simulink model "sm_tractor_row_crop"  (R2024b)
settings: Solver=ode23t  StartTime=0.0  StopTime=20  FixedStep=1/1000  MaxStep=0.2  RelTol=1e-3  AbsTol=1e-3  EnableMultiTasking=on
PostLoadFcn:
  | sm_tractor_row_crop_config_maneuver(bdroot,VehicleData,'stepsteer');
StartFcn:
  | tic
StopFcn:
  | Elapsed_Sim_Time = toc;
undefined symbols (not defined in the file): FL, FR, HMPST, InitVehicle, Maneuver, RL, RR, SceneData, targetSpeed, VehicleData, X, Y, Z
libraries: sm_lib x84, sm_vehicle_utilities_lib x40, fl_lib x15, nesl_utility x14, simulink x4, sm_tractor_row_crop_lib x3, sm_tractor_row_crop_lib_vnts x2, Tractor_Geometry x2, Driver_Long_Lat_Stanley x1, Maneuver_Get_Pose x1
(part 1 of 4)
CloseFcn:
  | try,close(h1_sm_vehicle_2axle_heave_roll),end
  | clear h1_sm_vehicle_2axle_heave_roll
  | try,close(h2_sm_vehicle_2axle_heave_roll),end
  | clear h2_sm_vehicle_2axle_heave_roll
  | try,close(h3_sm_vehicle_2axle_heave_roll),end
  | clear h3_sm_vehicle_2axle_heave_roll
  | 
  | 
  | clear simlog_sm_vehicle_2axle_heave_roll
  | clear logsout_sm_vehicle_2axle_heave_roll
Description:
  | Row Crop Tractor
  | 
  | Copyright 2022-2024 The MathWorks, Inc.
settings Model: Creator=smiller  LastModifiedBy=smiller
settings SolverCC: AutoScaleAbsTol=off  AlgebraicLoopSolver=TrustRegion
settings DataIOCC: SaveFormat=Array  SaveOutput=off  ReturnWorkspaceOutputs=off  SignalLoggingName=logsout_sm_tractor_row_crop  OutputTimes=[0:0.01:10]
settings OptimizationCC: ReuseModelBlockBuffer=off  ExpressionDepthLimit=2147483647  LifeSpan=inf
settings DebuggingCC: UnderspecifiedInitializationDetection=Classic  MergeDetectMultiDrivingBlocksExec=none  SolverPrmCheckMsg=warning  UnconnectedInputMsg=warning  UnconnectedOutputMsg=warning  UnconnectedLineMsg=warning  StateNameClashWarn=warning  PregeneratedLibrarySubsystemCodeDiagnostic=none  SFUnexpectedBacktrackingDiag=warning  SFNoUnconditionalDefaultTransitionDiag=warning  SFExecutionAtInitializationDiag=none  ArithmeticOperatorsInVariantConditions=warning
settings HardwareCC: ProdBitPerPointer=32  ProdBitPerSizeT=32  ProdBitPerPtrDiffT=32  ProdLargestAtomicFloat=None  ProdIntDivRoundTo=Undefined  ProdEndianess=Unspecified  ProdWordSize=32  ProdHWDeviceType=32-bit Generic
settings ModelReferenceCC: EnableRefExpFcnMdlSchedulingChecks=on  PropagateSignalLabelsOutOfModel=off
settings SFSimCC: SimUseLocalCustomCode=off  CustomCodeUndefinedFunction=UseInterfaceOnly
settings RTWCC: RTWUseLocalCustomCode=off  GPUComputeCapability=3.5  DLArmComputeVersion=19.05
settings CodeAppCC: StateflowObjectComments=on
settings GRTTargetCC: TargetLangStandard=C89/C90 (ANSI)
settings ConfigComp: CovMetricSettings=dw  CovSaveCumulativeToWorkspaceVar=on  CovSaveSingleToWorkspaceVar=on  CovExternalEMLEnable=off
settings SimscapeCC: SimscapeNormalizeSystem=off  SimscapeLogType=all  SimscapeLogToSDI=on  SimscapeLogName=simlog_sm_tractor_row_crop  SimscapeLogLimitData=off
settings ConfigurationSet: Description=SimMechanics 2G
settings DiagnosticsConfigSet: SimMechanicsUnconnectedFramePorts=none  SimMechanicsConflictingReferenceFrames=none
settings ExplorerConfigSet: InternalSimMechanicsExplorerSettings="<ExplorerConfiguration><canonicalview>default</canonicalview><AnimationSetting><BasePlaybackSpeed>1.0</BasePlaybackSpeed><PlaybackSpeedFactor>2.0</PlaybackSpeedFactor></AnimationSetting><TilePanel><TileInfo><Tiles Columns=\"2\" Count=\"3\" Rows=\"2\"><Column Weight=\"0.6147\"/><Column Weight=\"0.3853\"/><Row Weight=\"0.3693\"/><Row Weight=\"0.6307\"/><Tile Height=\"1\" Width=\"1\" X=\"0\" Y=\"0\"/><Tile Height=\"1\" Width=\"1\" X=\"0\" Y=\"1\"/><Tile Height=\"2\" Width=\"1\" X=\"1\" Y=\"0\"/></Tiles></TileInfo><SceneInfo><SceneViewer><BGColor><R>1</R><G>1</G><B>1</B></BGColor><Camera><DoPerspective>on</DoPerspective><Position><X>-1.49999999999999911</X><Y>1.54074395550978868e-32</Y><Z>10.6999999999999993</Z></Position><Center><X>-1.49999999999999911</X><Y>1.54074395550978868e-32</Y><Z>9.69999999999999929</Z></Center><Up><X>0</X><Y>1</Y><Z>0</Z></Up><ViewLimDist>1</ViewLimDist><YLim>0.466307658154998583</YLim><XLim>1.34838716914770518</XLim></Camera></SceneViewer><SceneViewer><BGColor><R>1</R><G>1</G><B>1</B></BGColor><Camera><DoPerspective>on</DoPerspective><Position><X>2.34000000000000163</X><Y>-3.20000000000000151</Y><Z>1.80000000000000004</Z></Position><Center><X>1.58973091910295716</X><Y>-2.57477576591913149</Y><Z>1.58507916953470085</Z></Center><Up><X>-0.16510675539218278</X><Y>0.137588962826818928</Y><Z>0.976631474319820447</Z></Up><ViewLimDist>1</ViewLimDist><YLim>0.466307658154998583</YLim><XLim>0.779836453951521791</XLim></Camera></SceneViewer><SceneViewer><BGColor><R>1</R><G>1</G><B>1</B></BGColor><Camera><DoPerspective>on</DoPerspective><Position><X>-6.5</X><Y>3.46944695195361419e-16</Y><Z>1.79999999999999982</Z></Position><Center><X>-5.52335553329491002</X><Y>3.46944695195361419e-16</Y><Z>1.58513821732488003</Z></Center><Up><X>0.214861782675119795</X><Y>-1.71056941445900502e-49</Y><Z>0.976644466705089975</Z></Up><ViewLimDist>1</ViewLimDist><YLim>0.466307658154998583</YLim><XLim>0.303969645724483983</XLim></Camera></SceneViewer></SceneInfo></TilePanel><MechEditorPanel><Cameras><Camera><Id>Camera1</Id><Value><Name>Track FixO FR</Name><NativeCamera><PositionTrackingFeature>Tractor.Camera_Frames.Frame_FixO_FR.R</PositionTrackingFeature><CenterTrackingFeature>Tractor.Camera_Frames.Frame_FixO_FR.R</CenterTrackingFeature><UpVectorTrackingFeature>Tractor.Camera_Frames.Frame_FixO_FR.R</UpVectorTrackingFeature><CenterTrackingOrigin>off</CenterTrackingOrigin><CenterTrackingDirection>+X</CenterTrackingDirection><UpVectorTrackingDirection>+Z</UpVectorTrackingDirection></NativeCamera></Value></Camera><Camera><Id>Camera2</Id><Value><Name>Track FixO Right</Name><NativeCamera><PositionTrackingFeature>Tractor.Camera_Frames.Frame_FixO_Right.R</PositionTrackingFeature><CenterTrackingFeature>Tractor.Camera_Frames.Frame_FixO_Right.R</CenterTrackingFeature><UpVectorTrackingFeature>Tractor.Camera_Frames.Frame_FixO_Right.R</UpVectorTrackingFeature><CenterTrackingOrigin>off</CenterTrackingOrigin><CenterTrackingDirection>+X</CenterTrackingDirection><UpVectorTrackingDirection>+Z</UpVectorTrackingDirection></NativeCamera></Value></Camera><Camera><Id>Camera3</Id><Value><Name>Track FixO RR</Name><NativeCamera><PositionTrackingFeature>Tractor.Camera_Frames.Frame_FixO_RR.R</PositionTrackingFeature><CenterTrackingFeature>Tractor.Camera_Frames.Frame_FixO_RR.R</CenterTrackingFeature><UpVectorTrackingFeature>Tractor.Camera_Frames.Frame_FixO_RR.R</UpVectorTrackingFeature><CenterTrackingOrigin>off</CenterTrackingOrigin><CenterTrackingDirection>+X</CenterTrackingDirection><UpVectorTrackingDirection>+Z</UpVectorTrackingDirection></NativeCamera></Value></Camera><Camera><Id>Camera4</Id><Value><Name>Track FixO RL</Name><NativeCamera><PositionTrackingFeature>Tractor.Camera_Frames.Frame_FixO_RL.R</PositionTrackingFeature><CenterTrackingFeature>Tractor.Camera_Frames.Frame_FixO_RL.R</CenterTrackingFeature><UpVectorTrackingFeature>Tractor.Camera_Frames.Frame_FixO_RL.R</UpVectorTrackingFeature><CenterTrackingOrigin>off</CenterTrackingOrigin><CenterTrackingDirection>+X</CenterTrackingDirection><UpVectorTrackingDirection>+Z</UpVectorTrackingDirection></NativeCamera></Value></Camera><Camera><Id>Camera5</Id><Value><Name>Track FixO Left</Name><NativeCamera><PositionTrackingFeature>Tractor.Camera_Frames.Frame_FixO_Left.R</PositionTrackingFeature><CenterTrackingFeature>Tractor.Camera_Frames.Frame_FixO_Left.R</CenterTrackingFeature><UpVectorTrackingFeature>Tractor.Camera_Frames.Frame_FixO_Left.R</UpVectorTrackingFeature><CenterTrackingOrigin>off</CenterTrackingOrigin><CenterTrackingDirection>+X</CenterTrackingDirection><UpVectorTrackingDirection>+Z</UpVectorTrackingDirection></NativeCamera></Value></Camera><Camera><Id>Camera6</Id><Value><Name>Track FixO FL</Name><NativeCamera><PositionTrackingFeature>Tractor.Camera_Frames.Frame_FixO_FL.R</PositionTrackingFeature><CenterTrackingFeature>Tractor.Camera_Frames.Frame_FixO_FL.R</CenterTrackingFeature><UpVectorTrackingFeature>Tractor.Camera_Frames.Frame_FixO_FL.R</UpVectorTrackingFeature><CenterTrackingOrigin>off</CenterTrackingOrigin><CenterTrackingDirection>+X</CenterTrackingDirection><UpVectorTrackingDirection>+Z</UpVectorTrackingDirection></NativeCamera></Value></Camera><Camera><Id>Camera7</Id><Value><Name>Track FixO Top</Name><NativeCamera><PositionTrackingFeature>Tractor.Camera_Frames.Frame_FixO_Top.R</PositionTrackingFeature><CenterTrackingFeature>Tractor.Camera_Frames.Frame_FixO_Top.R</CenterTrackingFeature><UpVectorTrackingFeature>Tractor.Camera_Frames.Frame_FixO_Top.R</UpVectorTrackingFeature><CenterTrackingOrigin>off</CenterTrackingOrigin><CenterTrackingDirection>+X</CenterTrackingDirection><UpVectorTrackingDirection>+Z</UpVectorTrackingDirection></NativeCamera></Value></Camera><Camera><Id>Camera8</Id><Value><Name>Track FixO Front</Name><NativeCamera><PositionTrackingFeature>Tractor.Camera_Frames.Frame_FixO_Front.R</PositionTrackingFeature><CenterTrackingFeature>Tractor.Camera_Frames.Frame_FixO_Front.R</CenterTrackingFeature><UpVectorTrackingFeature>Tractor.Camera_Frames.Frame_FixO_Front.R</UpVectorTrackingFeature><CenterTrackingOrigin>off</CenterTrackingOrigin><CenterTrackingDirection>+X</CenterTrackingDirection><UpVectorTrackingDirection>+Z</UpVectorTrackingDirection></NativeCamera></Value></Camera><Camera><Id>Camera9</Id><Value><Name>Track FixO Rear</Name><NativeCamera><PositionTrackingFeature>Tractor.Camera_Frames.Frame_FixO_Rear.R</PositionTrackingFeature><CenterTrackingFeature>Tractor.Camera_Frames.Frame_FixO_Rear.R</CenterTrackingFeature><UpVectorTrackingFeature>Tractor.Camera_Frames.Frame_FixO_Rear.R</UpVectorTrackingFeature><CenterTrackingOrigin>off</CenterTrackingOrigin><CenterTrackingDirection>+X</CenterTrackingDirection><UpVectorTrackingDirection>+Z</UpVectorTrackingDirection></NativeCamera></Value></Camera><Camera><Id>Camera10</Id><Value><Name>Track FR</Name><NativeCamera><PositionTrackingFeature>Tractor.Camera_Frames.Frame_FR.R</PositionTrackingFeature><CenterTrackingFeature>Tractor.Camera_Frames.Frame_FR.R</CenterTrackingFeature><UpVectorTrackingFeature>Tractor.Camera_Frames.Frame_FR.R</UpVectorTrackingFeature><CenterTrackingOrigin>off</CenterTrackingOrigin><CenterTrackingDirection>+X</CenterTrackingDirection><UpVectorTrackingDirection>+Z</UpVectorTrackingDirection></NativeCamera></Value></Camera><Camera><Id>Camera11</Id><Value><Name>Track Right</Name><NativeCamera><PositionTrackingFeature>Tractor.Camera_Frames.Frame_Right.R</PositionTrackingFeature><CenterTrackingFeature>Tractor.Camera_Frames.Frame_Right.R</CenterTrackingFeature><UpVectorTrackingFeature>Tractor.Camera_Frames.Frame_Right.R</UpVectorTrackingFeature><CenterTrackingOrigin>off</CenterTrackingOrigin><CenterTrackingDirection>+X</CenterTrackingDirection><UpVectorTrackingDirection>+Z</UpVectorTrackingDirection></NativeCamera></Value></Camera><Camera><Id>Camera12</Id><Value><Name>Track RR</Name><NativeCamera><PositionTrackingFeature>Tractor.Camera_Frames.Frame_RR.R</PositionTrackingFeature><CenterTrackingFeature>Tractor.Camera_Frames.Frame_RR.R</CenterTrackingFeature><UpVectorTrackingFeature>Tractor.Camera_Frames.Frame_RR.R</UpVectorTrackingFeature><CenterTrackingOrigin>off</CenterTrackingOrigin><CenterTrackingDirection>+X</CenterTrackingDirection><UpVectorTrackingDirection>+Z</UpVectorTrackingDirection></NativeCamera></Value></Camera><Camera><Id>Camera13</Id><Value><Name>Track RL</Name><NativeCamera><PositionTrackingFeature>Tractor.Camera_Frames.Frame_RL.R</PositionTrackingFeature><CenterTrackingFeature>Tractor.Camera_Frames.Frame_RL.R</CenterTrackingFeature><UpVectorTrackingFeature>Tractor.Camera_Frames.Frame_RL.R</UpVectorTrackingFeature><CenterTrackingOrigin>off</CenterTrackingOrigin><CenterTrackingDirection>+X</CenterTrackingDirection><UpVectorTrackingDirection>+Z</UpVectorTrackingDirection></NativeCamera></Value></Camera><Camera><Id>Camera14</Id><Value><Name>Track Left</Name><NativeCamera><PositionTrackingFeature>Tractor.Camera_Frames.Frame_Left.R</PositionTrackingFeature><CenterTrackingFeature>Tractor.Camera_Frames.Frame_Left.R</CenterTrackingFeature><UpVectorTrackingFeature>Tractor.Camera_Frames.Frame_Left.R</UpVectorTrackingFeature><CenterTrackingOrigin>off</CenterTrackingOrigin><CenterTrackingDirection>+X</CenterTrackingDirection><UpVectorTrackingDirection>+Z</UpVectorTrackingDirection></NativeCamera></Value></Camera><Camera><Id>Camera15</Id><Value><Name>Track FL</Name><NativeCamera><PositionTrackingFeature>Tractor.Camera_Frames.Frame_FL.R</PositionTrackingFeature><CenterTrackingFeature>Tractor.Camera_Frames.Frame_FL.R</CenterTrackingFeature><UpVectorTrackingFeature>Tractor.Camera_Frames.Frame_FL.R</UpVectorTrackingFeature><CenterTrackingOrigin>off</CenterTrackingOrigin><CenterTrackingDirection>+X</CenterTrackingDirection><UpVectorTrackingDirection>+Z</UpVectorTrackingDirection></NativeCamera></Value></Camera><Camera><Id>Camera16</Id><Value><Name>Track Top</Name><NativeCamera><PositionTrackingFeature>Tractor.Camera_Frames.Frame_Top.R</PositionTrackingFeature><CenterTrackingFeature>Tractor.Camera_Frames.Frame_Top.R</CenterTrackingFeature><UpVectorTrackingFeature>Tractor.Camera_Frames.Frame_Top.R</UpVectorTrackingFeature><CenterTrackingOrigin>off</CenterTrackingOrigin><CenterTrackingDirection>+X</CenterTrackingDirection><UpVectorTrackingDirection>+Z</UpVectorTrackingDirection></NativeCamera></Value></Camera><Camera><Id>Camera17</Id><Value><Name>Track Front</Name><NativeCamera><PositionTrackingFeature>Tractor.Camera_Frames.Frame_Front.R</PositionTrackingFeature><CenterTrackingFeature>Tractor.Camera_Frames.Frame_Front.R</CenterTrackingFeature><UpVectorTrackingFeature>Tractor.Camera_Frames.Frame_Front.R</UpVectorTrackingFeature><CenterTrackingOrigin>off</CenterTrackingOrigin><CenterTrackingDirection>+X</CenterTrackingDirection><UpVectorTrackingDirection>+Z</UpVectorTrackingDirection></NativeCamera></Value></Camera><Camera><Id>Camera18</Id><Value><Name>Track Rear</Name><NativeCamera><PositionTrackingFeature>Tractor.Camera_Frames.Frame_Rear.R</PositionTrackingFeature><CenterTrackingFeature>Tractor.Camera_Frames.Frame_Rear.R</CenterTrackingFeature><UpVectorTrackingFeature>Tractor.Camera_Frames.Frame_Rear.R</UpVectorTrackingFeature><CenterTrackingOrigin>off</CenterTrackingOrigin><CenterTrackingDirection>+X</CenterTrackingDirection><UpVectorTrackingDirection>+Z</UpVectorTrackingDirection></NativeCamera></Value></Camera><Camera><Id>Camera19</Id><Value><Name>Track SuspF</Name><NativeCamera><PositionTrackingFeature>Tractor.Camera_Frames.Frame_SuspF.R</PositionTrackingFeature><CenterTrackingFeature>Tractor.Camera_Frames.Frame_SuspF.R</CenterTrackingFeature><UpVectorTrackingFeature>Tractor.Camera_Frames.Frame_SuspF.R</UpVectorTrackingFeature><CenterTrackingOrigin>off</CenterTrackingOrigin><CenterTrackingDirection>+X</CenterTrackingDirection><UpVectorTrackingDirection>+Z</UpVectorTrackingDirection></NativeCamera></Value></Camera><Camera><Id>Camera20</Id><Value><Name>Track SuspR</Name><NativeCamera><PositionTrackingFeature>Tractor.Camera_Frames.Frame_SuspR.R</PositionTrackingFeature><CenterTrackingFeature>Tractor.Camera_Frames.Frame_SuspR.R</CenterTrackingFeature><UpVectorTrackingFeature>Tractor.Camera_Frames.Frame_SuspR.R</UpVectorTrackingFeature><CenterTrackingOrigin>off</CenterTrackingOrigin><CenterTrackingDirection>+X</CenterTrackingDirection><UpVectorTrackingDirection>+Z</UpVectorTrackingDirection></NativeCamera></Value></Camera><Camera><Id>Camera21</Id><Value><Name>Track WheelFR</Name><NativeCamera><PositionTrackingFeature>Tractor.Camera_Frames.Frame_Wheel_FR.R</PositionTrackingFeature><CenterTrackingFeature>Tractor.Camera_Frames.Frame_Wheel_FR.R</CenterTrackingFeature><UpVectorTrackingFeature>Tractor.Camera_Frames.Frame_Wheel_FR.R</UpVectorTrackingFeature><CenterTrackingOrigin>off</CenterTrackingOrigin><CenterTrackingDirection>+X</CenterTrackingDirection><UpVectorTrackingDirection>+Z</UpVectorTrackingDirection></NativeCamera></Value></Camera><Camera><Id>Camera22</Id><Value><Name>Track WheelRR</Name><NativeCamera><PositionTrackingFeature>Tractor.Camera_Frames.Frame_Wheel_RR.R</PositionTrackingFeature><CenterTrackingFeature>Tractor.Camera_Frames.Frame_Wheel_RR.R</CenterTrackingFeature><UpVectorTrackingFeature>Tractor.Camera_Frames.Frame_Wheel_RR.R</UpVectorTrackingFeature><CenterTrackingOrigin>off</CenterTrackingOrigin><CenterTrackingDirection>+X</CenterTrackingDirection><UpVectorTrackingDirection>+Z</UpVectorTrackingDirection></NativeCamera></Value></Camera><Camera><Id>Camera23</Id><Value><Name>Track WheelRL</Name><NativeCamera><PositionTrackingFeature>Tractor.Camera_Frames.Frame_Wheel_RL.R</PositionTrackingFeature><CenterTrackingFeature>Tractor.Camera_Frames.Frame_Wheel_RL.R</CenterTrackingFeature><UpVectorTrackingFeature>Tractor.Camera_Frames.Frame_Wheel_RL.R</UpVectorTrackingFeature><CenterTrackingOrigin>off</CenterTrackingOrigin><CenterTrackingDirection>+X</CenterTrackingDirection><UpVectorTrackingDirection>+Z</UpVectorTrackingDirection></NativeCamera></Value></Camera><Camera><Id>Camera24</Id><Value><Name>Track WheelFL</Name><NativeCamera><PositionTrackingFeature>Tractor.Camera_Frames.Frame_Wheel_FL.R</PositionTrackingFeature><CenterTrackingFeature>Tractor.Camera_Frames.Frame_Wheel_FL.R</CenterTrackingFeature><UpVectorTrackingFeature>Tractor.Camera_Frames.Frame_Wheel_FL.R</UpVectorTrackingFeature><CenterTrackingOrigin>off</CenterTrackingOrigin><CenterTrackingDirection>+X</CenterTrackingDirection><UpVectorTrackingDirection>+Z</UpVectorTrackingDirection></NativeCamera></Value></Camera><Camera><Id>Camera25</Id><Value><Name>View Seat FL</Name><NativeCamera><PositionTrackingFeature>Tractor.Camera_Frames.Frame_View_Seat_FL.R</PositionTrackingFeature><CenterTrackingFeature>Tractor.Camera_Frames.Frame_View_Seat_FL.R</CenterTrackingFeature><UpVectorTrackingFeature>Tractor.Camera_Frames.Frame_View_Seat_FL.R</UpVectorTrackingFeature><CenterTrackingOrigin>off</CenterTrackingOrigin><CenterTrackingDirection>+X</CenterTrackingDirection><UpVectorTrackingDirection>+Z</UpVectorTrackingDirection></NativeCamera></Value></Camera><Camera><Id>Camera26</Id><Value><Name>View Seat FR</Name><NativeCamera><PositionTrackingFeature>Tractor.Camera_Frames.Frame_View_Seat_FR.R</PositionTrackingFeature><CenterTrackingFeature>Tractor.Camera_Frames.Frame_View_Seat_FR.R</CenterTrackingFeature><UpVectorTrackingFeature>Tractor.Camera_Frames.Frame_View_Seat_FR.R</UpVectorTrackingFeature><CenterTrackingOrigin>off</CenterTrackingOrigin><CenterTrackingDirection>+X</CenterTrackingDirection><UpVectorTrackingDirection>+Z</UpVectorTrackingDirection></NativeCamera></Value></Camera><Camera><Id>Camera27</Id><Value><Name>View Susp FR</Name><NativeCamera><PositionTrackingFeature>Tractor.Camera_Frames.Frame_View_Susp_FR.R</PositionTrackingFeature><CenterTrackingFeature>Tractor.Camera_Frames.Frame_View_Susp_FR.R</CenterTrackingFeature><UpVectorTrackingFeature>Tractor.Camera_Frames.Frame_View_Susp_FR.R</UpVectorTrackingFeature><CenterTrackingOrigin>off</CenterTrackingOrigin><CenterTrackingDirection>+X</CenterTrackingDirection><UpVectorTrackingDirection>+Z</UpVectorTrackingDirection></NativeCamera></Value></Camera><Camera><Id>Camera28</Id><Value><Name>View Susp RR</Name><NativeCamera><PositionTrackingFeature>Tractor.Camera_Frames.Frame_View_Susp_RR.R</PositionTrackingFeature><CenterTrackingFeature>Tractor.Camera_Frames.Frame_View_Susp_RR.R</CenterTrackingFeature><UpVectorTrackingFeature>Tractor.Camera_Frames.Frame_View_Susp_RR.R</UpVectorTrackingFeature><CenterTrackingOrigin>off</CenterTrackingOrigin><CenterTrackingDirection>+X</CenterTrackingDirection><UpVectorTrackingDirection>+Z</UpVectorTrackingDirection></NativeCamera></Value></Camera><Camera><Id>Camera29</Id><Value><Name>View Susp RL</Name><NativeCamera><PositionTrackingFeature>Tractor.Camera_Frames.Frame_View_Susp_RL.R</PositionTrackingFeature><CenterTrackingFeature>Tractor.Camera_Frames.Frame_View_Susp_RL.R</CenterTrackingFeature><UpVectorTrackingFeature>Tractor.Camera_Frames.Frame_View_Susp_RL.R</UpVectorTrackingFeature><CenterTrackingOrigin>off</CenterTrackingOrigin><CenterTrackingDirection>+X</CenterTrackingDirection><UpVectorTrackingDirection>+Z</UpVectorTrackingDirection></NativeCamera></Value></Camera><Camera><Id>Camera30</Id><Value><Name>View Susp FL</Name><NativeCamera><PositionTrackingFeature>Tractor.Camera_Frames.Frame_View_Susp_FL.R</PositionTrackingFeature><CenterTrackingFeature>Tractor.Camera_Frames.Frame_View_Susp_FL.R</CenterTrackingFeature><UpVectorTrackingFeature>Tractor.Camera_Frames.Frame_View_Susp_FL.R</UpVectorTrackingFeature><CenterTrackingOrigin>off</CenterTrackingOrigin><CenterTrackingDirection>+X</CenterTrackingDirection><UpVectorTrackingDirection>+Z</UpVectorTrackingDirection></NativeCamera></Value></Camera><Camera><Id>Camera31</Id><Value><Name>Dolly Camera</Name><NativeCamera><PositionTrackingFeature>Tractor.Camera_Frames.Frame_Dolly.R</PositionTrackingFeature><CenterTrackingFeature>Tractor.Camera_Frames.Frame_Dolly.R</CenterTrackingFeature><UpVectorTrackingFeature>Tractor.Camera_Frames.Frame_Dolly.R</UpVectorTrackingFeature><CenterTrackingOrigin>off</CenterTrackingOrigin><CenterTrackingDirection>+X</CenterTrackingDirection><UpVectorTrackingDirection>+Z</UpVectorTrackingDirection></NativeCamera></Value></Camera><Camera><Id>Camera32</Id><Value><Name>Track Dolly Camera</Name><NativeCamera><PositionTrackingFeature>Tractor.Camera_Frames.Frame_Dolly.R</PositionTrackingFeature><CenterTrackingFeature>Tractor.Camera_Frames.Transform_Camera_Ref.F</CenterTrackingFeature><UpVectorTrackingFeature>Tractor.Camera_Frames.World_Frame.W</UpVectorTrackingFeature><CenterTrackingOrigin>on</CenterTrackingOrigin><UpVectorTrackingDirection>+Z</UpVectorTrackingDirection></NativeCamera></Value></Camera></Cameras><GfxPanelCameraMap><MapElement CameraMLId=\"Camera7\" GfxPanelIndex=\"0\"/><MapElement CameraMLId=\"Camera1\" GfxPanelIndex=\"1\"/><MapElement CameraMLId=\"Camera9\" GfxPanelIndex=\"2\"/></GfxPanelCameraMap><VideoCreator><PlaybackSpeedRatio>1.0</PlaybackSpeedRatio><FrameRate>30</FrameRate><VideoFormat>MPEG-4</VideoFormat><FrameSize>[800 450]</FrameSize></VideoCreator></MechEditorPanel></ExplorerConfiguration>"

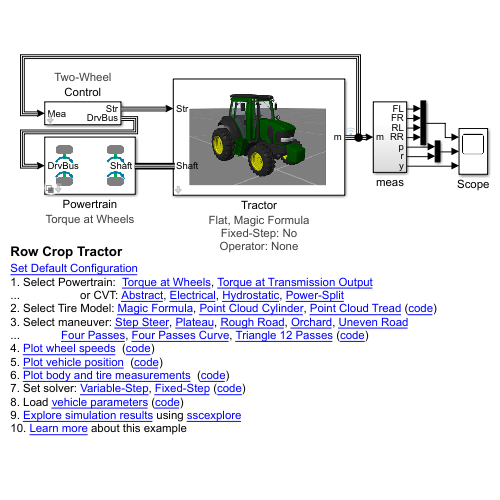
[thumbnail: Simulink's stored preview of the top-level diagram]
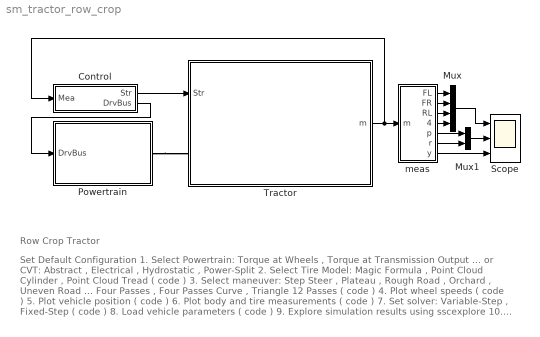
== system sm_tractor_row_crop ==
  note: Row Crop Tractor
  note: Set Default Configuration
      | 1. Select Powertrain: Torque at Wheels , Torque at Transmission Output
      | ... or CVT: Abstract , Electrical , Hydrostatic , Power-Split
      | 2. Select Tire Model: Magic Formula , Point Cloud Cylinder , Point Cloud Tread ( code )
      | 3. Select maneuver: Step Steer , Plateau , Rough Road , Orchard , Uneven Road
      | ... Four Passes , Four Passes Curve , Triangle 12 Passes ( code )
      | 4. Plot wheel speeds ( code )
      | 5. Plot vehicle position ( code )
      | 6. Plot body and tire measurements ( code )
      | 7. Set solver: Variable-Step , Fixed-Step ( code )
      | 8. Load vehicle parameters ( code )
      | 9. Explore simulation results using sscexplore
      | 10. Learn more about this example
  Control : Subsystem  mask{popup_steer_control=Step Steer (open loop), popup_steer_mode=Two-Wheel}
      mask prompts: popup_steer_control "Steer Control"; popup_steer_mode "Steer Mode"
      mask init:
      | switch popup_steer_control
      |     case 1
      |         set_param([gcb '/Steering'],'LabelModeActiveChoice','Closed_Loop')
      |     case 2
      |         set_param([gcb '/Steering'],'LabelModeActiveChoice','Step_Steer')
      |     case 3
      |         set_param([gcb '/Steering'],'LabelModeActiveChoice','No_Steer')
      |     case 4
      |         set_param([gcb '/Steering'],'LabelModeActiveChoice','Interactive')
      | end
      settings: AttributesFormatString=%<popup_steer_mode>
      mask TypeOptions popup_steer_mode: Two-Wheel | Proportional | True Track | Crab | Delay | None
  Mux : Mux
  Mux1 : Mux  Inputs=2
  Powertrain : Subsystem  Variant=on  VariantControlMode=label  VariantControl=Powertrain  LabelModeActiveChoice=Torque4  mask{popup_powertrain_config=Torque at Wheels}
      mask prompts: popup_powertrain_config "Powertrain Configuration"
      mask init:
      | blk_h = gcb;
      | switch(get_param(blk_h,'popup_powertrain_config'))
      |     case('Torque at Wheels')
      |         set_param(blk_h,'LabelModeActiveChoice','Torque4');
      |     case('Torque at Transmission Output')
      |         set_param(blk_h,'LabelModeActiveChoice','Torque1');
      |     case('CVT Abstract')
      |         set_param(blk_h,'LabelModeActiveChoice','CVT');
      |         set_param([blk_h '/CVT/Transmission'],'LabelModeActiveChoice','Abstract');
      |     case('CVT Electrical')
      |         set_param(blk_h,'LabelModeActiveChoice','CVT');
      |         set_param([blk_h '/CVT/Transmission'],'LabelModeActiveChoice','Electrical');
      |     case('CVT Hydrostatic')
      |         set_param(blk_h,'LabelModeActiveChoice','CVT');
      |         set_param([blk_h '/CVT/Transmission'],'LabelModeActiveChoice','Hydrostatic');
      |     case('CVT Power Split HM')
      |         set_param(blk_h,'LabelModeActiveChoice','CVT');
      |         set_param([blk_h '/CVT/Transmission'],'LabelModeActiveChoice','Power_Split_HM');
      | end
      settings: AttributesFormatString=%<popup_powertrain_config>
      mask TypeOptions popup_powertrain_config: Torque at Wheels | Torque at Transmission Output | CVT Abstract | CVT Electrical | CVT Hydrostatic | CVT Power Split HM
  Scope : Scope  NumInputPorts=3
  Tractor : Subsystem  mask(Vehicle and Scene){vehdata=VehicleData, initveh=InitVehicle, popup_road_surface=Flat, popup_tire_type=Magic Formula, popup_local_solver=No, popup_operator=None}
      mask prompts: vehdata "Vehicle Data (structure)"; initveh "Initial Position, Velocity (structure)"; popup_road_surface "Road Surface"; popup_tire_type "Tire Model"; popup_local_solver "Fixed-Step Simulation"; popup_operator "Operator Type"
      mask help: Models a vehicle with a configurable scene. Vehicle parameters are defined within a single data structure. A separate data structure defines the initial position, orientation, and speed of the vehicle and the wheels.
      mask init:
      | bh = gcb;
      | surface_name = strrep(get_param(bh,'popup_road_surface'),' ','_');
      | set_param([bh '/Scene'],'LabelModeActiveChoice',surface_name);
      | 
      | tire_type = strrep(get_param(bh,'popup_tire_type'),' ','_');
      | set_param([bh '/Wheel FL'],'LabelModeActiveChoice',tire_type);
      | set_param([bh '/Wheel FR'],'LabelModeActiveChoice',tire_type);
      | set_param([bh '/Wheel RL'],'LabelModeActiveChoice',tire_type);
      | set_param([bh '/Wheel RR'],'LabelModeActiveChoice',tire_type);
      | 
      | if(strcmp(get_param(bh,'popup_local_solver'),'Yes'))
      |     set_param([bh '/World'],'DoFixedCost','on','UseLocalSolver','on')
      | else
      |     set_param([bh '/World'],'DoFixedCost','off','UseLocalSolver','off')
      | end
      settings: AttributesFormatString=|
      | %<popup_road_surface>, %<popup_tire_type>
      | Fixed-Step: %<popup_local_solver>
      | Operator: %<popup_operator>
      mask TypeOptions popup_road_surface: Flat | Plateau | Rough Road | Orchard | Uneven Road
      mask TypeOptions popup_tire_type: Magic Formula | Point Cloud
      mask TypeOptions popup_local_solver: No | Yes
      mask TypeOptions popup_operator: Body/popup_operator
      mask Display: image('sm_tractor_row_crop_grid.png');
  meas : Subsystem
  wires:
  Control/1(Str) -> Tractor/1(Str)
  Tractor/1(m) -> Control/1(Mea), meas/1(m)
  Mux/1 -> Scope/1
  meas/1(FL) -> Mux/1
  meas/2(FR) -> Mux/2
  meas/3(RL) -> Mux/3
  meas/4(RR) -> Mux/4
  meas/5(p) -> Mux1/1
  meas/6(r) -> Mux1/2
  Mux1/1 -> Scope/2
  meas/7(y) -> Scope/3
  Control/2(DrvBus) -> Powertrain/1(DrvBus)
  connections:
  Powertrain/RConn1 -- Tractor/LConn1

== system sm_tractor_row_crop/Control ==
  BusElementIn1 : Inport  PortName=Mea
  Bus Creator : BusCreator  Inputs=2
  Bus Selector1 : BusSelector  OutputSignals=aSteerWheel
  Mode : Constant  Value=popup_steer_mode
  Prop Steer Rear : Constant  Value=0.8
  Scope : Scope
  Steer Mode : Subsystem
  Steering : Subsystem  Variant=on  VariantControlMode=label  VariantControl=Steering  LabelModeActiveChoice=Step_Steer
  Str : Outport
  DrvBus : Outport  Port=2
  wires:
  BusElementIn1/1 -> Steering/1(VehBus)
  Steer Mode/1(Str) -> Str/1
  Bus Selector1/1 -> Scope/1  "<aSteerWheel>"
  Bus Creator/1 -> Steer Mode/1(Ctrl)
  Mode/1 -> Bus Creator/1  "Mode"
  Prop Steer Rear/1 -> Bus Creator/2  "propR"
  Steering/1(DrvBus) -> Bus Selector1/1, DrvBus/1, Steer Mode/2(Drv)

== system sm_tractor_row_crop/Powertrain ==
  DrvBus : Inport
  CVT : Subsystem  VariantControl=CVT
      mask Display: image('sm_tractor_row_crop_powertrain_cvt.png')
  Torque1 : Subsystem  VariantControl=Torque1  mask{checkbox_torque_source=on}
      mask prompts: checkbox_torque_source "Enable Torque Source"
      mask Display: image('sm_tractor_row_crop_powertrain_torque1.png')
  Torque4 : Subsystem  VariantControl=Torque4  mask{checkbox_torque_source=on, vehSpdCmd=InitVehicle.Vehicle.vx}
      mask prompts: checkbox_torque_source "Enable Torque Source"; vehSpdCmd "Target Speed (m/s)"
      mask Display: image('sm_tractor_row_crop_powertrain_torque4.png')
  Shaft : PMIOPort  Side=Right

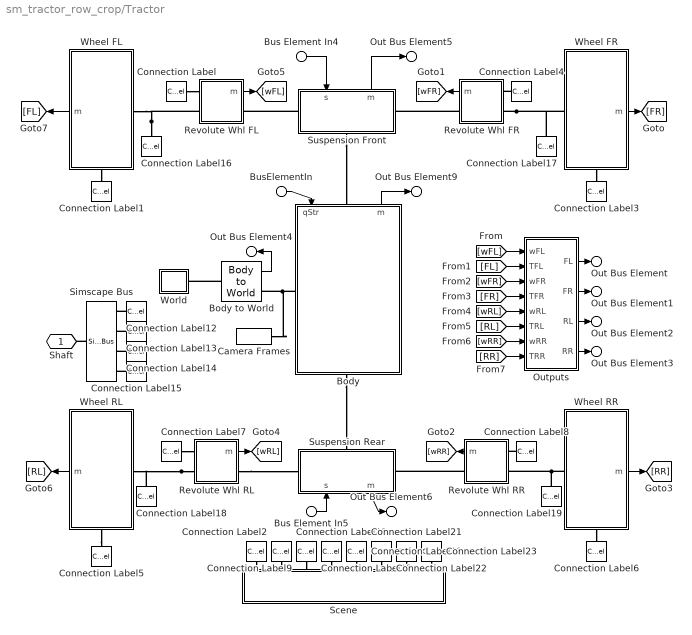
== system sm_tractor_row_crop/Tractor ==
  Bus Element In4 : Inport  PortName=Str  Element=qWhlF
  Bus Element In5 : Inport  PortName=Str  Element=qWhlR
  BusElementIn : Inport  PortName=Str  Element=aSteerWheel
  Body : Subsystem  mask{xRefToFA=vehdata.Body.FA, xRefToRA=vehdata.Body.RA, xyzRefToCG=vehdata.Body.CG, mBody=vehdata.Body.Mass, JBody=vehdata.Body.Inertias, clrBody=vehdata.Body.Color, opcBody=vehdata.Body.Opacity, popup_operator=None}
      mask prompts: xRefToFA "Offset Reference to Front Axle (m)"; xRefToRA "Offset Reference to Rear Axle (m)"; xyzRefToCG "Offset Reference to CG [x y z] (m)"; mBody "Body Mass (kg)"; JBody "Body Inertia [Ixx Iyy Izz] (kg*m^2)"; clrBody "Body Color [R G B]"; opcBody "Body Opacity (0-1)"; popup_operator "Operator Type"
      settings: PortSchema="{\"entries\":[{\"content\":{\"sides\":[{\"content\":{\"connectorIds\":[\"LConn1\"]},\"type\":\"ConnectorPlacement.EquallySpacedRectSide\",\"uuid\":\"96da581a-446c-43fa-8064-b9be639c090a\"},{\"content\":{\"connectorIds\":[\"Out1\",\"RConn1\",\"In1\"],\"side\":\"RIGHT\"},\"type\":\"ConnectorPlacement.EquallySpacedRectSide\",\"uuid\":\"2c5988da-ae00-48b3-be94-fd9e5696b9c8\"},{\"content\":{\"side\":\"TOP\"},\"type\":\"ConnectorPlacement.EquallySpacedRectSide\",\"uuid\":\"77344741-9809-4470-a690-faf7ab180986\"},{\"content\":{\"connectorIds\":[\"RConn2\"],\"side\":\"BOTTOM\"},\"type\":\"ConnectorPlacement.EquallySpacedRectSide\",\"uuid\":\"18f3e2d3-f6ed-4015-9148-fd9a3ca5738a\"}]},\"type\":\"ConnectorPlacement.EquallySpacedConnector\",\"uuid\":\"db176424-9696-4c3b-8300-543540a9ef25\"}],\"packageUris\":[\"http://schema.mathworks.com/mf0/Connector/R2020b\"],\"version\":\"1.0\"}"
      mask TypeOptions popup_operator: Operator/popup_operator
      mask Display: image('sm_tractor_row_crop_body.png');
  Body to World : sm_vehicle_utilities_lib/Body to World  Init=initveh.Vehicle  SpecifyPosTarget=on
  Camera Frames : sm_vehicle_utilities_lib/Camera Frames  Camera=Camera  popup_dolly_camera=Off
  Connection Label : ConnectionLabel  Label=FL
  Connection Label1 : ConnectionLabel  Label=GFL
  Connection Label10 : ConnectionLabel  Label=GRL
  Connection Label11 : ConnectionLabel  Label=GRR
  Connection Label12 : ConnectionLabel  Label=FL
  Connection Label13 : ConnectionLabel  Label=FR
  Connection Label14 : ConnectionLabel  Label=RL
  Connection Label15 : ConnectionLabel  Label=RR
  Connection Label16 : ConnectionLabel  Label=RFL
  Connection Label17 : ConnectionLabel  Label=RFR
  Connection Label18 : ConnectionLabel  Label=RRL
  Connection Label19 : ConnectionLabel  Label=RRR
  Connection Label2 : ConnectionLabel  Label=GFL
  Connection Label20 : ConnectionLabel  Label=RFL
  Connection Label21 : ConnectionLabel  Label=RFR
  Connection Label22 : ConnectionLabel  Label=RRL
  Connection Label23 : ConnectionLabel  Label=RRR
  Connection Label3 : ConnectionLabel  Label=GFR
  Connection Label4 : ConnectionLabel  Label=FR
  Connection Label5 : ConnectionLabel  Label=GRL
  Connection Label6 : ConnectionLabel  Label=GRR
  Connection Label7 : ConnectionLabel  Label=RL
  Connection Label8 : ConnectionLabel  Label=RR
  Connection Label9 : ConnectionLabel  Label=GFR
  Outputs : Subsystem
  Revolute Whl FL : Subsystem
  Revolute Whl FR : Subsystem
  Revolute Whl RL : Subsystem
  Revolute Whl RR : Subsystem
  Scene : Subsystem  Variant=on  VariantControlMode=label  VariantControl=Scene  LabelModeActiveChoice=Flat
      settings: AttributesFormatString=%<LabelModeActiveChoice>
      mask Display: disp(' ')
  Simscape Bus : SimscapeBus  HierarchyStrings=FL;FR;RL;RR
  Suspension Front : Subsystem  mask(Suspension with Heave, Roll, and Ackerman Steering){zHeave=vehdata.SuspF.Heave.Height, kHeave=vehdata.SuspF.Heave.Stiffness, dHeave=vehdata.SuspF.Heave.Damping, xEqHeave=vehdata.SuspF.Heave.EqPos, zRoll=vehdata.SuspF.Roll.Height, kRoll=vehdata.SuspF.Roll.Stiffness, dRoll=vehdata.SuspF.Roll.Damping, aEqRoll=vehdata.SuspF.Roll.EqPos, mUnsprungMass=vehdata.SuspF.UnsprungMass.Mass, JUnsprungMass=vehdata.SuspF.UnsprungMass.Inertia, zUnsprungMass=vehdata.SuspF.UnsprungMass.Height, rUnsprungMass=vehdata.SuspF.UnsprungMass.Radius, lUnsprungMass=vehdata.SuspF.UnsprungMass.Length, zHub=vehdata.SuspF.Hub.Height, yTrack=vehdata.SuspF.Track, wheelbase=sum(abs(vehdata.Body.RA-vehdata.Body.FA)), steerRatio=vehdata.SuspF.SteerRatio}
      mask prompts: zHeave "Height (m)"; kHeave "Stiffness (N/m)"; dHeave "Damping (N/(m/s))"; xEqHeave "Equilibrium Position (m)"; zRoll "Height (m)"; kRoll "Stiffness (N*m/rad)"; dRoll "Damping (N*m/(rad/s)"; aEqRoll "Equilibrium Position (rad)"; mUnsprungMass "Mass (kg)"; JUnsprungMass "Inertia (kg*m^2)"; zUnsprungMass "Height (m)"; rUnsprungMass "Radius (m)"; lUnsprungMass "Length (m)"; zHub "Wheel Center Height (m)"; yTrack "Track Width (m)"; steerRatio "Steering Ratio"
      mask help: Models a suspension with heave and roll degrees of freedom for a single axle, with Ackermann steering. All heights are measured relative to the bottom of the wheels.
      settings: PortSchema="{\"entries\":[{\"content\":{\"sides\":[{\"content\":{\"connectorIds\":[\"LConn1\"]},\"type\":\"ConnectorPlacement.EquallySpacedRectSide\",\"uuid\":\"0af81f34-82de-4f02-a8a7-ec45be82faea\"},{\"content\":{\"connectorIds\":[\"In1\",\"Out1\"],\"side\":\"RIGHT\"},\"type\":\"ConnectorPlacement.EquallySpacedRectSide\",\"uuid\":\"9bc48957-2707-4e2f-b988-a5743aaf8f58\"},{\"content\":{\"connectorIds\":[\"LConn2\"],\"side\":\"TOP\"},\"type\":\"ConnectorPlacement.EquallySpacedRectSide\",\"uuid\":\"08055243-2fee-46c8-8a4b-df5231c2978e\"},{\"content\":{\"connectorIds\":[\"RConn1\"],\"side\":\"BOTTOM\"},\"type\":\"ConnectorPlacement.EquallySpacedRectSide\",\"uuid\":\"745b1e5c-9113-4e99-a394-3eadcd3cd6f8\"}]},\"type\":\"ConnectorPlacement.EquallySpacedConnector\",\"uuid\":\"5011d399-f081-425d-a1fb-c00f3859766f\"}],\"packageUris\":[\"http://schema.mathworks.com/mf0/Connector/R2020b\"],\"version\":\"1.0\"}"
      mask DialogControl cont_heave_roll Prompt: Heave, Roll
      mask DialogControl group_heave Prompt: Heave
      mask DialogControl group_roll Prompt: Roll
      mask DialogControl cont_unsprung_mass Prompt: Unsprung Mass
      mask DialogControl cont_wheels_steering Prompt: Wheels, Steering
  Suspension Rear : Subsystem  mask(Suspension with Heave, Roll, and Ackerman Steering){zHeave=vehdata.SuspR.Heave.Height, kHeave=vehdata.SuspR.Heave.Stiffness, dHeave=vehdata.SuspR.Heave.Damping, xEqHeave=vehdata.SuspR.Heave.EqPos, zRoll=vehdata.SuspR.Roll.Height, kRoll=vehdata.SuspR.Roll.Stiffness, dRoll=vehdata.SuspR.Roll.Damping, aEqRoll=vehdata.SuspR.Roll.EqPos, mUnsprungMass=vehdata.SuspR.UnsprungMass.Mass, JUnsprungMass=vehdata.SuspR.UnsprungMass.Inertia, zUnsprungMass=vehdata.SuspR.UnsprungMass.Height, rUnsprungMass=vehdata.SuspR.UnsprungMass.Radius, lUnsprungMass=vehdata.SuspR.UnsprungMass.Length, zHub=vehdata.SuspR.Hub.Height, yTrack=vehdata.SuspR.Track, wheelbase=sum(abs(vehdata.Body.RA-vehdata.Body.FA)), steerRatio=vehdata.SuspR.SteerRatio}
      mask prompts: zHeave "Height (m)"; kHeave "Stiffness (N/m)"; dHeave "Damping (N/(m/s))"; xEqHeave "Equilibrium Position (m)"; zRoll "Height (m)"; kRoll "Stiffness (N*m/rad)"; dRoll "Damping (N*m/(rad/s)"; aEqRoll "Equilibrium Position (rad)"; mUnsprungMass "Mass (kg)"; JUnsprungMass "Inertia (kg*m^2)"; zUnsprungMass "Height (m)"; rUnsprungMass "Radius (m)"; lUnsprungMass "Length (m)"; zHub "Wheel Center Height (m)"; yTrack "Track Width (m)"; steerRatio "Steering Ratio"
      mask help: Models a suspension with heave and roll degrees of freedom for a single axle, with Ackermann steering. All heights are measured relative to the bottom of the wheels.
      settings: PortSchema="{\"entries\":[{\"content\":{\"sides\":[{\"content\":{\"connectorIds\":[\"LConn1\"]},\"type\":\"ConnectorPlacement.EquallySpacedRectSide\",\"uuid\":\"0af81f34-82de-4f02-a8a7-ec45be82faea\"},{\"content\":{\"connectorIds\":[\"In1\",\"Out1\"],\"side\":\"RIGHT\"},\"type\":\"ConnectorPlacement.EquallySpacedRectSide\",\"uuid\":\"9bc48957-2707-4e2f-b988-a5743aaf8f58\"},{\"content\":{\"connectorIds\":[\"LConn2\"],\"side\":\"TOP\"},\"type\":\"ConnectorPlacement.EquallySpacedRectSide\",\"uuid\":\"08055243-2fee-46c8-8a4b-df5231c2978e\"},{\"content\":{\"connectorIds\":[\"RConn1\"],\"side\":\"BOTTOM\"},\"type\":\"ConnectorPlacement.EquallySpacedRectSide\",\"uuid\":\"745b1e5c-9113-4e99-a394-3eadcd3cd6f8\"}]},\"type\":\"ConnectorPlacement.EquallySpacedConnector\",\"uuid\":\"5011d399-f081-425d-a1fb-c00f3859766f\"}],\"packageUris\":[\"http://schema.mathworks.com/mf0/Connector/R2020b\"],\"version\":\"1.0\"}"
      mask DialogControl cont_heave_roll Prompt: Heave, Roll
      mask DialogControl group_heave Prompt: Heave
      mask DialogControl group_roll Prompt: Roll
      mask DialogControl cont_unsprung_mass Prompt: Unsprung Mass
      mask DialogControl cont_wheels_steering Prompt: Wheels, Steering
  Wheel FL : Subsystem  Variant=on  VariantControlMode=label  VariantControl=Wheel FL  LabelModeActiveChoice=Magic_Formula
      settings: PortSchema="{\"entries\":[{\"content\":{\"sides\":[{\"content\":{\"connectorIds\":[\"LConn1\"]},\"type\":\"ConnectorPlacement.EquallySpacedRectSide\",\"uuid\":\"a5957755-4b21-43b1-b34a-d64340a2a9fa\"},{\"content\":{\"connectorIds\":[\"Out1\"],\"side\":\"RIGHT\"},\"type\":\"ConnectorPlacement.EquallySpacedRectSide\",\"uuid\":\"7abc4e22-bce4-4e01-bde2-484a70cd2d65\"},{\"content\":{\"side\":\"TOP\"},\"type\":\"ConnectorPlacement.EquallySpacedRectSide\",\"uuid\":\"bb9080de-8600-4afc-aa18-a9613af8dea2\"},{\"content\":{\"connectorIds\":[\"RConn1\"],\"side\":\"BOTTOM\"},\"type\":\"ConnectorPlacement.EquallySpacedRectSide\",\"uuid\":\"dc1ddff3-45d7-4df4-bcab-c75e74c98592\"}]},\"type\":\"ConnectorPlacement.EquallySpacedConnector\",\"uuid\":\"8576f11d-c6ed-476d-923e-0f1bd6b3d66d\"}],\"packageUris\":[\"http://schema.mathworks.com/mf0/Connector/R2020b\"],\"version\":\"1.0\"}"
  Wheel FR : Subsystem  Variant=on  VariantControlMode=label  VariantControl=Wheel FR  LabelModeActiveChoice=Magic_Formula
      settings: PortSchema="{\"entries\":[{\"content\":{\"sides\":[{\"content\":{\"connectorIds\":[\"LConn1\"]},\"type\":\"ConnectorPlacement.EquallySpacedRectSide\",\"uuid\":\"a5957755-4b21-43b1-b34a-d64340a2a9fa\"},{\"content\":{\"connectorIds\":[\"Out1\"],\"side\":\"RIGHT\"},\"type\":\"ConnectorPlacement.EquallySpacedRectSide\",\"uuid\":\"7abc4e22-bce4-4e01-bde2-484a70cd2d65\"},{\"content\":{\"side\":\"TOP\"},\"type\":\"ConnectorPlacement.EquallySpacedRectSide\",\"uuid\":\"bb9080de-8600-4afc-aa18-a9613af8dea2\"},{\"content\":{\"connectorIds\":[\"RConn1\"],\"side\":\"BOTTOM\"},\"type\":\"ConnectorPlacement.EquallySpacedRectSide\",\"uuid\":\"dc1ddff3-45d7-4df4-bcab-c75e74c98592\"}]},\"type\":\"ConnectorPlacement.EquallySpacedConnector\",\"uuid\":\"8576f11d-c6ed-476d-923e-0f1bd6b3d66d\"}],\"packageUris\":[\"http://schema.mathworks.com/mf0/Connector/R2020b\"],\"version\":\"1.0\"}"
  Wheel RL : Subsystem  Variant=on  VariantControlMode=label  VariantControl=Wheel RL  LabelModeActiveChoice=Magic_Formula
      settings: PortSchema="{\"entries\":[{\"content\":{\"sides\":[{\"content\":{\"connectorIds\":[\"LConn1\"]},\"type\":\"ConnectorPlacement.EquallySpacedRectSide\",\"uuid\":\"a5957755-4b21-43b1-b34a-d64340a2a9fa\"},{\"content\":{\"connectorIds\":[\"Out1\"],\"side\":\"RIGHT\"},\"type\":\"ConnectorPlacement.EquallySpacedRectSide\",\"uuid\":\"7abc4e22-bce4-4e01-bde2-484a70cd2d65\"},{\"content\":{\"side\":\"TOP\"},\"type\":\"ConnectorPlacement.EquallySpacedRectSide\",\"uuid\":\"bb9080de-8600-4afc-aa18-a9613af8dea2\"},{\"content\":{\"connectorIds\":[\"RConn1\"],\"side\":\"BOTTOM\"},\"type\":\"ConnectorPlacement.EquallySpacedRectSide\",\"uuid\":\"dc1ddff3-45d7-4df4-bcab-c75e74c98592\"}]},\"type\":\"ConnectorPlacement.EquallySpacedConnector\",\"uuid\":\"8576f11d-c6ed-476d-923e-0f1bd6b3d66d\"}],\"packageUris\":[\"http://schema.mathworks.com/mf0/Connector/R2020b\"],\"version\":\"1.0\"}"
  Wheel RR : Subsystem  Variant=on  VariantControlMode=label  VariantControl=Wheel RR  LabelModeActiveChoice=Magic_Formula
      settings: PortSchema="{\"entries\":[{\"content\":{\"sides\":[{\"content\":{\"connectorIds\":[\"LConn1\"]},\"type\":\"ConnectorPlacement.EquallySpacedRectSide\",\"uuid\":\"a5957755-4b21-43b1-b34a-d64340a2a9fa\"},{\"content\":{\"connectorIds\":[\"Out1\"],\"side\":\"RIGHT\"},\"type\":\"ConnectorPlacement.EquallySpacedRectSide\",\"uuid\":\"7abc4e22-bce4-4e01-bde2-484a70cd2d65\"},{\"content\":{\"side\":\"TOP\"},\"type\":\"ConnectorPlacement.EquallySpacedRectSide\",\"uuid\":\"bb9080de-8600-4afc-aa18-a9613af8dea2\"},{\"content\":{\"connectorIds\":[\"RConn1\"],\"side\":\"BOTTOM\"},\"type\":\"ConnectorPlacement.EquallySpacedRectSide\",\"uuid\":\"dc1ddff3-45d7-4df4-bcab-c75e74c98592\"}]},\"type\":\"ConnectorPlacement.EquallySpacedConnector\",\"uuid\":\"8576f11d-c6ed-476d-923e-0f1bd6b3d66d\"}],\"packageUris\":[\"http://schema.mathworks.com/mf0/Connector/R2020b\"],\"version\":\"1.0\"}"
  World : Subsystem  mask{DoFixedCost=off, UseLocalSolver=off, LocalSolverSampleTime=1/1000}
      mask TypeOptions DoFixedCost:
      | Solver
      | Configuration/DoFixedCost
      mask TypeOptions UseLocalSolver:
      | Solver
      | Configuration/UseLocalSolver
      mask TypeOptions LocalSolverSampleTime:
      | Solver
      | Configuration/LocalSolverSampleTime
  Shaft : PMIOPort  Side=Left
  Out Bus Element9 : Outport  PortName=m  Element=Chassis
  Out Bus Element : Outport  PortName=m  Element=TireFL
  Out Bus Element1 : Outport  PortName=m  Element=TireFR
  Out Bus Element2 : Outport  PortName=m  Element=TireRL
  Out Bus Element3 : Outport  PortName=m  Element=TireRR
  Out Bus Element4 : Outport  PortName=m  Element=World
  Out Bus Element5 : Outport  PortName=m  Element=SuspF
  Out Bus Element6 : Outport  PortName=m  Element=SuspR
  wires:
  Bus Element In4/1 -> Suspension Front/1(s)
  Revolute Whl FR/1(m) -> [wFR]
  Body/1(m) -> Out Bus Element9/1
  [wFL] -> Outputs/1(wFL)
  [FL] -> Outputs/2(TFL)
  Outputs/1(FL) -> Out Bus Element/1
  [wFR] -> Outputs/3(wFR)
  [FR] -> Outputs/4(TFR)
  [wRL] -> Outputs/5(wRL)
  [RL] -> Outputs/6(TRL)
  [wRR] -> Outputs/7(wRR)
  [RR] -> Outputs/8(TRR)
  Outputs/2(FR) -> Out Bus Element1/1
  Outputs/3(RL) -> Out Bus Element2/1
  Outputs/4(RR) -> Out Bus Element3/1
  Body to World/1 -> Out Bus Element4/1
  Suspension Front/1(m) -> Out Bus Element5/1
  Suspension Rear/1(m) -> Out Bus Element6/1
  Bus Element In5/1 -> Suspension Rear/1(s)
  Revolute Whl FL/1(m) -> [wFL]
  Revolute Whl RL/1(m) -> [wRL]
  Revolute Whl RR/1(m) -> [wRR]
  BusElementIn/1 -> Body/1(qStr)
  Wheel FL/1(m) -> [FL]
  Wheel FR/1(m) -> [FR]
  Wheel RL/1(m) -> [RL]
  Wheel RR/1(m) -> [RR]
  connections:
  Body to World/LConn1 -- World/RConn1
  Revolute Whl FR/RConn1 -- Suspension Front/RConn1
  Revolute Whl RL/RConn1 -- Suspension Rear/LConn2
  Revolute Whl RR/RConn1 -- Suspension Rear/RConn1
  Camera Frames/RConn1 -- Body/RConn2 -- Body to World/RConn1
  Suspension Front/LConn1 -- Body/RConn1
  Body/LConn1 -- Suspension Rear/LConn1
  Suspension Front/LConn2 -- Revolute Whl FL/RConn1
  Connection Label/LConn1 -- Revolute Whl FL/LConn1
  Connection Label4/LConn1 -- Revolute Whl FR/LConn1
  Connection Label7/LConn1 -- Revolute Whl RL/LConn1
  Connection Label8/LConn1 -- Revolute Whl RR/LConn1
  Connection Label12/LConn1 -- Simscape Bus/LConn1
  Connection Label13/LConn1 -- Simscape Bus/LConn2
  Connection Label14/LConn1 -- Simscape Bus/LConn3
  Connection Label15/LConn1 -- Simscape Bus/LConn4
  Simscape Bus/RConn1 -- Shaft/RConn1
  Connection Label2/LConn1 -- Scene/LConn1
  Connection Label9/LConn1 -- Scene/LConn2
  Connection Label10/LConn1 -- Scene/LConn3
  Connection Label11/LConn1 -- Scene/LConn4
  Connection Label20/LConn1 -- Scene/LConn5
  Connection Label21/LConn1 -- Scene/LConn6
  Connection Label22/LConn1 -- Scene/LConn7
  Connection Label23/LConn1 -- Scene/LConn8
  Connection Label16/LConn1 -- Revolute Whl FL/LConn2 -- Wheel FL/LConn1
  Wheel FL/RConn1 -- Connection Label1/LConn1
  Revolute Whl FR/LConn2 -- Connection Label17/LConn1 -- Wheel FR/LConn1
  Wheel FR/RConn1 -- Connection Label3/LConn1
  Revolute Whl RL/LConn2 -- Connection Label18/LConn1 -- Wheel RL/LConn1
  Wheel RL/RConn1 -- Connection Label5/LConn1
  Connection Label19/LConn1 -- Revolute Whl RR/LConn2 -- Wheel RR/LConn1
  Wheel RR/RConn1 -- Connection Label6/LConn1

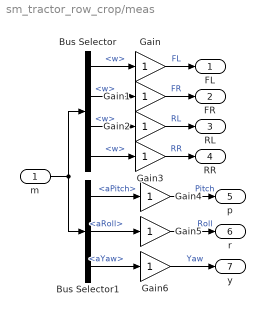
== system sm_tractor_row_crop/meas ==
  m : Inport
  Bus Selector : BusSelector  OutputSignals=TireFL.w,TireFR.w,TireRL.w,TireRR.w
  Bus Selector1 : BusSelector  OutputSignals=Chassis.Body.CG.aPitch,Chassis.Body.CG.aRoll,World.aYaw
  Gain{,1..6} (7 alike) : Gain
  FL : Outport
  FR : Outport  Port=2
  RL : Outport  Port=3
  RR : Outport  Port=4
  p : Outport  Port=5
  r : Outport  Port=6
  y : Outport  Port=7
  wires:
  Bus Selector/4 -> Gain3/1  "<w>"
  Bus Selector/2 -> Gain1/1  "<w>"
  Bus Selector/3 -> Gain2/1  "<w>"
  Bus Selector/1 -> Gain/1  "<w>"
  m/1 -> Bus Selector/1, Bus Selector1/1
  Gain3/1 -> RR/1  "RR"
  Gain/1 -> FL/1  "FL"
  Gain1/1 -> FR/1  "FR"
  Gain2/1 -> RL/1  "RL"
  Bus Selector1/1 -> Gain4/1  "<aPitch>"
  Bus Selector1/2 -> Gain5/1  "<aRoll>"
  Bus Selector1/3 -> Gain6/1  "<aYaw>"
  Gain6/1 -> y/1  "Yaw"
  Gain5/1 -> r/1  "Roll"
  Gain4/1 -> p/1  "Pitch"

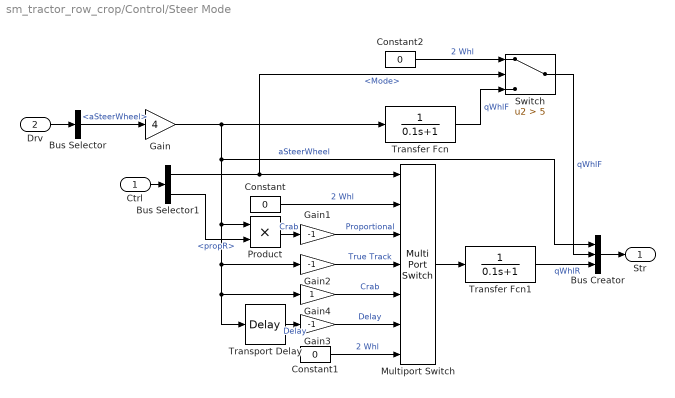
== system sm_tractor_row_crop/Control/Steer Mode ==
  Ctrl : Inport
  Drv : Inport  Port=2
  Bus Creator : BusCreator  Inputs=3
  Bus Selector : BusSelector  OutputSignals=aSteerWheel
  Bus Selector1 : BusSelector  OutputSignals=Mode,propR
  Constant : Constant  Value=0
  Constant1 : Constant  Value=0
  Constant2 : Constant  Value=0
  Gain : Gain  Gain=4
  Gain1 : Gain  Gain=-1
  Gain2 : Gain  Gain=-1
  Gain3 : Gain  Gain=-1
  Gain4 : Gain
  Multiport Switch : MultiPortSwitch  Inputs=6  SaturateOnIntegerOverflow=off  InputSameDT=off
  Product : Product
  Switch : Switch  Criteria=u2 > Threshold  Threshold=5  ZeroCross=off  SaturateOnIntegerOverflow=off  InputSameDT=off
  Transfer Fcn : TransferFcn  Denominator=[0.1 1]
  Transfer Fcn1 : TransferFcn  Denominator=[0.1 1]
  Transport Delay : TransportDelay  DelayTime=2  BufferSize=3072
  Str : Outport
  wires:
  Gain4/1 -> Multiport Switch/5  "Crab"
  Transport Delay/1 -> Gain3/1  "Delay"
  Multiport Switch/1 -> Transfer Fcn1/1
  Switch/1 -> Bus Creator/2  "qWhlF"
  Bus Creator/1 -> Str/1
  Gain2/1 -> Multiport Switch/4  "True Track"
  Gain1/1 -> Multiport Switch/3  "Proportional"
  Ctrl/1 -> Bus Selector1/1
  Bus Selector1/1 -> Switch/2, Multiport Switch/1  "<Mode>"
  Bus Selector1/2 -> Product/2  "<propR>"
  Bus Selector/1 -> Gain/1  "<aSteerWheel>"
  Transfer Fcn1/1 -> Bus Creator/3  "qWhlR"
  Product/1 -> Gain1/1  "Crab"
  Constant/1 -> Multiport Switch/2  "2 Whl"
  Gain3/1 -> Multiport Switch/6  "Delay"
  Drv/1 -> Bus Selector/1
  Constant1/1 -> Multiport Switch/7  "2 Whl"
  Transfer Fcn/1 -> Switch/3  "qWhlF"
  Constant2/1 -> Switch/1  "2 Whl"
  Gain/1 -> Transfer Fcn/1, Bus Creator/1, Product/1, Transport Delay/1, Gain4/1, Gain2/1  "aSteerWheel"

== system sm_tractor_row_crop/Control/Steering ==
  VehBus : Inport
  Closed Loop : Subsystem  VariantControl=Closed_Loop
  Interactive : Subsystem  VariantControl=Interactive  mask{Kp=4, Ki=0.1}
      mask prompts: Kp "Speed Control, Kp"; Ki "Speed Control, Ki"
  No Steer : Subsystem  VariantControl=No_Steer  mask{Kp=4, Ki=0.1}
      mask prompts: Kp "Speed Control, Kp"; Ki "Speed Control, Ki"
  Step Steer : Subsystem  VariantControl=Step_Steer  mask{Kp=4, Ki=0.1}
      mask prompts: Kp "Speed Kp"; Ki "Speed Ki"
  DrvBus : Outport
